simulink library "pilotlib"  (Simulink 8.8)
settings: Solver=VariableStepAuto  StartTime=0.0  StopTime=10.0  RelTol=1e-3
settings Model: SuppressorTable=22 serialization::archive 11 0 3 0 0 0 11 0  Creator=sven  LastModifiedBy=peyam

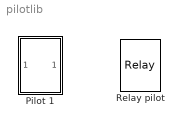
== system pilotlib ==
  Pilot 1 : Subsystem
  Relay pilot : Relay  OffSwitchValue=-eps  OnOutputValue=0.2  OffOutputValue=-0.2

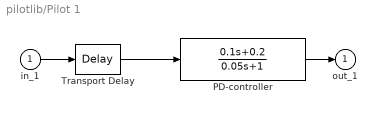
== system pilotlib/Pilot 1 ==
  in_1 : Inport
  PD-controller : TransferFcn  Numerator=[0.1 0.2]  Denominator=[0.05 1]
  Transport Delay : TransportDelay  DelayTime=0.3
  out_1 : Outport  InitialOutput=0
  wires:
  PD-controller/1 -> out_1/1
  Transport Delay/1 -> PD-controller/1
  in_1/1 -> Transport Delay/1
